simulink model "RegolazioneLQ_observer_mdl"  (Simulink 7.2)
settings: Solver=ode45  StartTime=0.0  StopTime=10.0  RelTol=1e-3
values from neighbouring files (symbols this model uses):
  C1 = [1 -1 0 0]    [TSC150918ProvaMatlab.m]
  Dx0 = [0.05 0.01 0 0]'    [TSC150918ProvaMatlab.m]
  L = - acker(A',C1',Po)'    [TSC150918ProvaMatlab.m]
undefined symbols (not defined in the file or in its folder): A, B, C, K
settings Model: Creator=lbiagiotti  LastModifiedBy=lbiagiotti

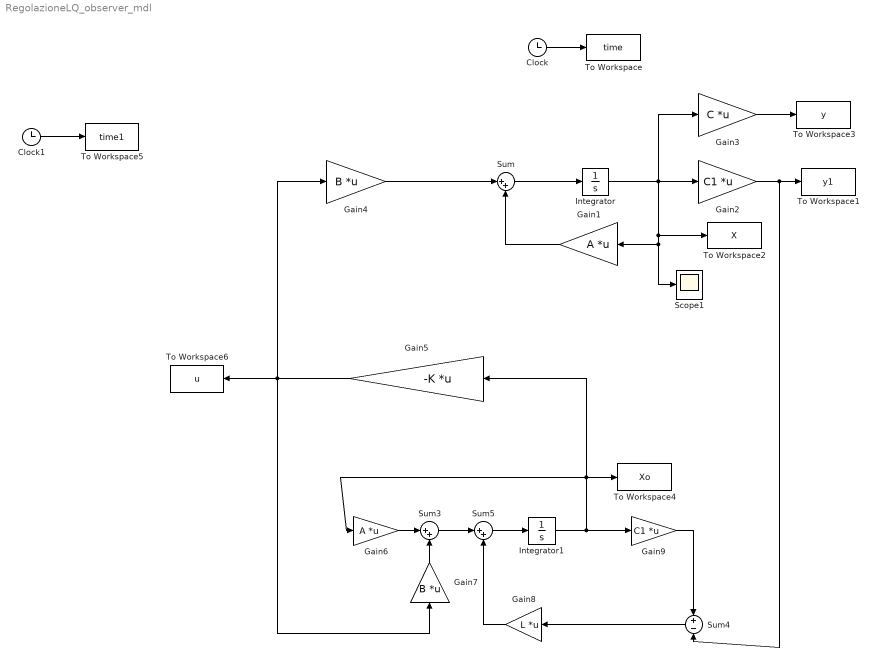
== system RegolazioneLQ_observer_mdl ==
  Clock : Clock
      settings: Decimation=10
  Clock1 : Clock
      settings: Decimation=10
  Gain1 : Gain  Orientation=left  Gain=A  Multiplication=Matrix(K*u)  ParameterDataType=sfix(16)  ParameterScaling=2^0  OutDataType=sfix(16)  OutScaling=2^0
  Gain2 : Gain  Gain=C1  Multiplication=Matrix(K*u)  ParameterDataType=sfix(16)  ParameterScaling=2^0  OutDataType=sfix(16)  OutScaling=2^0
  Gain3 : Gain  Gain=C  Multiplication=Matrix(K*u)  ParameterDataType=sfix(16)  ParameterScaling=2^0  OutDataType=sfix(16)  OutScaling=2^0
  Gain4 : Gain  Gain=B  Multiplication=Matrix(K*u)  ParameterDataType=sfix(16)  ParameterScaling=2^0  OutDataType=sfix(16)  OutScaling=2^0
  Gain5 : Gain  Orientation=left  Gain=-K  Multiplication=Matrix(K*u)  ParameterDataType=sfix(16)  ParameterScaling=2^0  OutDataType=sfix(16)  OutScaling=2^0
  Gain6 : Gain  Gain=A  Multiplication=Matrix(K*u)  ParameterDataType=sfix(16)  ParameterScaling=2^0  OutDataType=sfix(16)  OutScaling=2^0
  Gain7 : Gain  Orientation=up  Gain=B  Multiplication=Matrix(K*u)  ParameterDataType=sfix(16)  ParameterScaling=2^0  OutDataType=sfix(16)  OutScaling=2^0
  Gain8 : Gain  Orientation=left  Gain=L  Multiplication=Matrix(K*u)  ParameterDataType=sfix(16)  ParameterScaling=2^0  OutDataType=sfix(16)  OutScaling=2^0
  Gain9 : Gain  Gain=C1  Multiplication=Matrix(K*u)  ParameterDataType=sfix(16)  ParameterScaling=2^0  OutDataType=sfix(16)  OutScaling=2^0
  Integrator : Integrator  InitialCondition=Dx0
  Integrator1 : Integrator  InitialCondition=[0 0 0 0]
  Scope1 : Scope
  Sum : Sum  Inputs=|++  OutDataType=sfix(16)  OutScaling=2^0
  Sum3 : Sum  Inputs=|++  OutDataType=sfix(16)  OutScaling=2^0
  Sum4 : Sum  Orientation=left  Inputs=+-  OutDataType=sfix(16)  OutScaling=2^0
  Sum5 : Sum  Inputs=|++  OutDataType=sfix(16)  OutScaling=2^0
  To Workspace : ToWorkspace  VariableName=time  SampleTime=-1  SaveFormat=Array
  To Workspace1 : ToWorkspace  VariableName=y1  SampleTime=-1  SaveFormat=Array
  To Workspace2 : ToWorkspace  VariableName=X  SampleTime=-1  SaveFormat=Array
  To Workspace3 : ToWorkspace  VariableName=y  SampleTime=-1  SaveFormat=Array
  To Workspace4 : ToWorkspace  VariableName=Xo  SampleTime=-1  SaveFormat=Array
  To Workspace5 : ToWorkspace  VariableName=time1  SampleTime=-1  SaveFormat=Array
  To Workspace6 : ToWorkspace  VariableName=u  SampleTime=-1  SaveFormat=Array
  wires:
  Gain1/1 -> Sum/2
  Sum/1 -> Integrator/1
  Integrator/1 -> Gain2/1, To Workspace2/1, Gain1/1, Scope1/1, Gain3/1
  Clock/1 -> To Workspace/1
  Gain2/1 -> To Workspace1/1, Sum4/2
  Gain4/1 -> Sum/1
  Gain5/1 -> Gain4/1, Gain7/1, To Workspace6/1
  Gain6/1 -> Sum3/1
  Integrator1/1 -> Gain9/1, Gain6/1, To Workspace4/1, Gain5/1
  Gain7/1 -> Sum3/2
  Sum4/1 -> Gain8/1
  Gain8/1 -> Sum5/2
  Sum3/1 -> Sum5/1
  Sum5/1 -> Integrator1/1
  Gain9/1 -> Sum4/1
  Gain3/1 -> To Workspace3/1
  Clock1/1 -> To Workspace5/1
